simulink model "Width1"  (R2017b)
settings: Solver=FixedStepDiscrete  StartTime=0.0  StopTime=100  FixedStep=0.200000  RelTol=1e-3  EnableMultiTasking=on
undefined symbols (not defined in the file): pp_lib, SineWaveFunction
settings Model: Creator=hbourbou  LastModifiedBy=hbourbou
settings DataIOCC: ExternalInput=input_dataset  LimitDataPoints=on  SaveState=on
settings OptimizationCC: LifeSpan=inf
settings DebuggingCC: AlgebraicLoopMsg=error  ArtificialAlgebraicLoopMsg=error  SFUnexpectedBacktrackingDiag=warning  SFNoUnconditionalDefaultTransitionDiag=warning  SFExecutionAtInitializationDiag=none
settings HardwareCC: ProdBitPerPointer=32  ProdBitPerSizeT=32  ProdBitPerPtrDiffT=32  ProdLargestAtomicFloat=None  ProdIntDivRoundTo=Undefined  ProdEndianess=Unspecified  ProdWordSize=32  ProdHWDeviceType=32-bit Generic
settings ModelReferenceCC: PropagateSignalLabelsOutOfModel=off
settings CodeAppCC: StateflowObjectComments=on
settings GRTTargetCC: TargetLangStandard=C89/C90 (ANSI)  GeneratePreprocessorConditionals=Disable all  ExtMode=on
settings ConfigComp: CovMetricSettings=dw  CovHtmlReporting=on  CovSaveCumulativeToWorkspaceVar=on  CovSaveSingleToWorkspaceVar=on  CovExternalEMLEnable=off

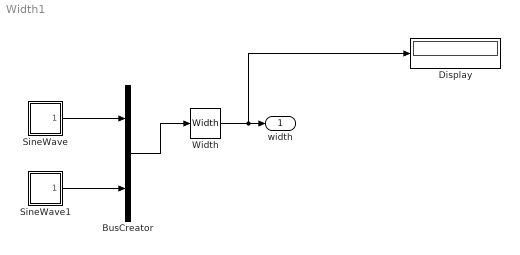
== system Width1 ==
  BusCreator : BusCreator  Inputs=2
  Display : Display
  SineWave : Subsystem  AncestorBlock=pp_lib/SineWaveFunction  TreatAsAtomicUnit=on
  SineWave1 : Subsystem  AncestorBlock=pp_lib/SineWaveFunction  TreatAsAtomicUnit=on
  Width : Width  DataType=uint8
  width : Outport
  wires:
  Width/1 -> Display/1, width/1
  SineWave/1(Out1) -> BusCreator/1
  SineWave1/1(Out1) -> BusCreator/2
  BusCreator/1 -> Width/1

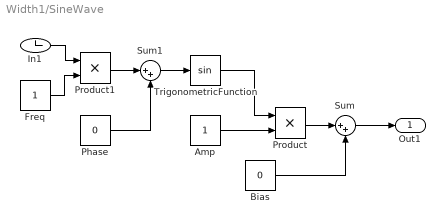
== system Width1/SineWave ==
  Amp : Constant
  Bias : Constant  Value=0
  Freq : Constant
  In1 : Clock
  Phase : Constant  Value=0
  Product : Product
  Product1 : Product
  Sum : Sum  Inputs=|++
  Sum1 : Sum  Inputs=|++
  TrigonometricFunction : Trigonometry
  Out1 : Outport
  wires:
  Freq/1 -> Product1/2
  Phase/1 -> Sum1/2
  Sum1/1 -> TrigonometricFunction/1
  Product1/1 -> Sum1/1
  In1/1 -> Product1/1
  Amp/1 -> Product/2
  TrigonometricFunction/1 -> Product/1
  Product/1 -> Sum/1
  Bias/1 -> Sum/2
  Sum/1 -> Out1/1

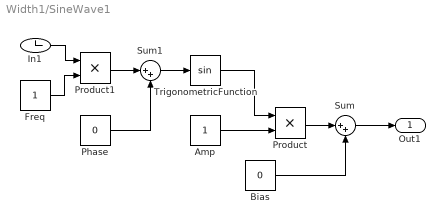
== system Width1/SineWave1 ==
  Amp : Constant
  Bias : Constant  Value=0
  Freq : Constant
  In1 : Clock
  Phase : Constant  Value=0
  Product : Product
  Product1 : Product
  Sum : Sum  Inputs=|++
  Sum1 : Sum  Inputs=|++
  TrigonometricFunction : Trigonometry
  Out1 : Outport
  wires:
  Freq/1 -> Product1/2
  Phase/1 -> Sum1/2
  Sum1/1 -> TrigonometricFunction/1
  Product1/1 -> Sum1/1
  In1/1 -> Product1/1
  Amp/1 -> Product/2
  TrigonometricFunction/1 -> Product/1
  Product/1 -> Sum/1
  Bias/1 -> Sum/2
  Sum/1 -> Out1/1
